simulink subsystem "matrix_for_each_sref"  (R2024b)
settings: Solver=VariableStepAuto  StartTime=0.0  StopTime=10.0  RelTol=1e-3
libraries: hdlsllib x4
settings Model: Creator=aherrman  LastModifiedBy=aherrman

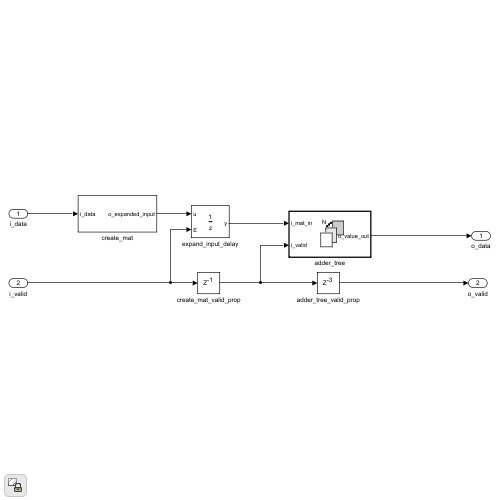
[thumbnail: Simulink's stored preview of the top-level diagram]
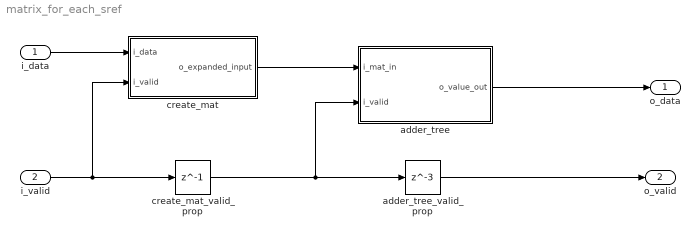
== system matrix_for_each_sref ==
  i_data : Inport
  i_valid : Inport  Port=2
  adder_tree : Subsystem  TreatAsAtomicUnit=on
  adder_tree_valid_prop : Delay  DelayLength=3
  create_mat : Subsystem
  create_mat_valid_prop : Delay  DelayLength=1
  o_data : Outport
  o_valid : Outport  Port=2
  wires:
  adder_tree/1(o_value_out) -> o_data/1
  create_mat/1(o_expanded_input) -> adder_tree/1(i_mat_in)
  i_data/1 -> create_mat/1(i_data)
  i_valid/1 -> create_mat_valid_prop/1, create_mat/2(i_valid)
  create_mat_valid_prop/1 -> adder_tree_valid_prop/1, adder_tree/2(i_valid)
  adder_tree_valid_prop/1 -> o_valid/1

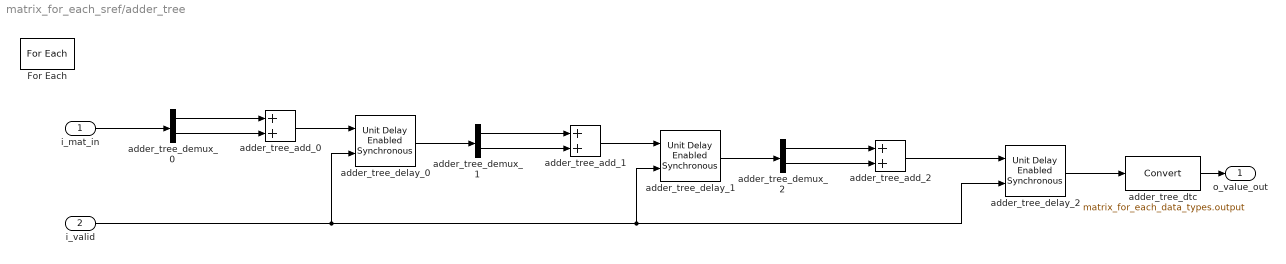
== system matrix_for_each_sref/adder_tree ==
  i_mat_in : Inport  Partition=on  PartitionDimension=1  PartitionWidth=1  PartitionOffset=0
  i_valid : Inport  Port=2
  For Each : ForEach  DisableCoverage=on
  adder_tree_add_0 : Sum
  adder_tree_add_1 : Sum
  adder_tree_add_2 : Sum
  adder_tree_delay_0 : hdlsllib/Discrete/Unit Delay Enabled Synchronous  InitialCondition=0.0  SampleTime=-1
  adder_tree_delay_1 : hdlsllib/Discrete/Unit Delay Enabled Synchronous  InitialCondition=0.0  SampleTime=-1
  adder_tree_delay_2 : hdlsllib/Discrete/Unit Delay Enabled Synchronous  InitialCondition=0.0  SampleTime=-1
  adder_tree_demux_0 : Demux  Outputs=2
  adder_tree_demux_1 : Demux  Outputs=2
  adder_tree_demux_2 : Demux  Outputs=2
  adder_tree_dtc : DataTypeConversion  OutDataTypeStr=matrix_for_each_data_types.output  SaturateOnIntegerOverflow=off  RndMeth=Floor
  o_value_out : Outport  ConcatenationDimension=1
  wires:
  i_valid/1 -> adder_tree_delay_0/2, adder_tree_delay_2/2, adder_tree_delay_1/2
  adder_tree_dtc/1 -> o_value_out/1
  adder_tree_delay_2/1 -> adder_tree_dtc/1
  adder_tree_add_2/1 -> adder_tree_delay_2/1
  adder_tree_delay_1/1 -> adder_tree_demux_2/1
  adder_tree_demux_2/2 -> adder_tree_add_2/2
  adder_tree_demux_2/1 -> adder_tree_add_2/1
  adder_tree_delay_0/1 -> adder_tree_demux_1/1
  adder_tree_add_1/1 -> adder_tree_delay_1/1
  adder_tree_demux_1/2 -> adder_tree_add_1/2
  adder_tree_demux_1/1 -> adder_tree_add_1/1
  adder_tree_add_0/1 -> adder_tree_delay_0/1
  i_mat_in/1 -> adder_tree_demux_0/1
  adder_tree_demux_0/2 -> adder_tree_add_0/2
  adder_tree_demux_0/1 -> adder_tree_add_0/1

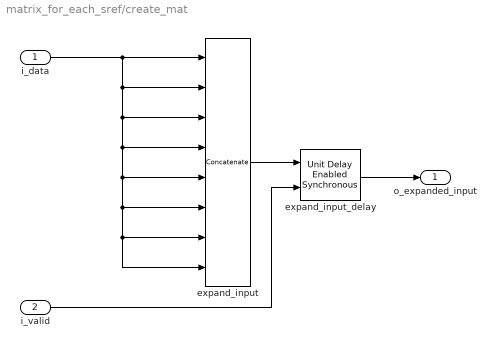
== system matrix_for_each_sref/create_mat ==
  i_data : Inport
  i_valid : Inport  Port=2
  expand_input : Concatenate  NumInputs=8  Mode=Multidimensional array  ConcatenateDimension=2
  expand_input_delay : hdlsllib/Discrete/Unit Delay Enabled Synchronous  InitialCondition=0.0  SampleTime=-1
  o_expanded_input : Outport
  wires:
  i_valid/1 -> expand_input_delay/2
  expand_input_delay/1 -> o_expanded_input/1
  expand_input/1 -> expand_input_delay/1
  i_data/1 -> expand_input/5, expand_input/6, expand_input/7, expand_input/8, expand_input/4, expand_input/3, expand_input/2, expand_input/1
